simulink model "LQR_Model"  (R2023b)
settings: Solver=VariableStepAuto  StartTime=0.0  StopTime=10.0  RelTol=1e-3
values from neighbouring files (symbols this model uses):
  A_mat = [0 0 1 0;0 0 0 1;0 (b*d)/(E) (-(c*G)/E) 0 ; 0 ((a*d)/E) (-b*G)/E 0 ]    [LQR.m]    (also in matlab.mat = [0 0 0 0 0 0 16.4102446308 112.769220168 1 0 2.36879708342 2)
  B_mat = [0;0;(c)*(H);(b)*(H)]    [LQR.m]    (also in matlab.mat = [0 0 152.465167276 137.218650549])
  C_mat = [1 0 0 0 ; 0 1 0 0]    [LQR.m]    (also in matlab.mat = [1  0  0  0; 0  1  0  0])
  k = lqr(A_mat,B_mat,Q,R)    [LQR.m]    (also in matlab.mat = [-0.316227766017 614.603053164 -26.5092676997 65.1532424468])
settings Model: Creator=peter  LastModifiedBy=peter

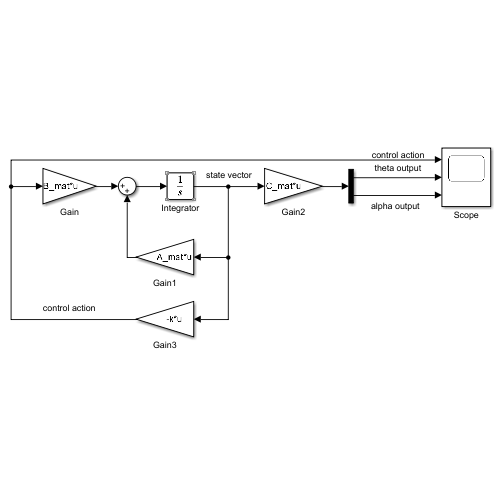
[thumbnail: Simulink's stored preview of the top-level diagram]
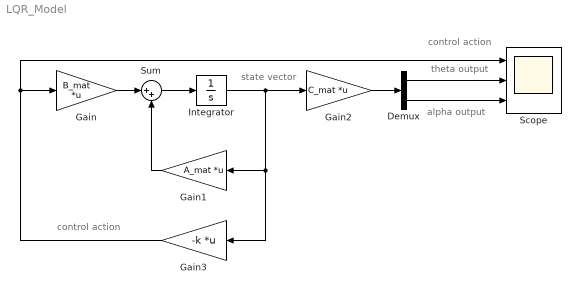
== system LQR_Model ==
  note: control action
  note: theta output
  note: alpha output
  note: state vector
  note: control action
  Demux : Demux  Outputs=2
  Gain : Gain  Gain=B_mat  Multiplication=Matrix(K*u)
  Gain1 : Gain  Gain=A_mat  Multiplication=Matrix(K*u)
  Gain2 : Gain  Gain=C_mat  Multiplication=Matrix(K*u)
  Gain3 : Gain  Gain=-k  Multiplication=Matrix(K*u)
  Integrator : Integrator  InitialCondition=[0.5 0.436 0 0]
  Scope : Scope  NumInputPorts=3
  Sum : Sum  Inputs=|++
  wires:
  Gain/1 -> Sum/1
  Sum/1 -> Integrator/1
  Integrator/1 -> Gain3/1, Gain1/1, Gain2/1
  Gain1/1 -> Sum/2
  Gain3/1 -> Gain/1, Scope/1
  Gain2/1 -> Demux/1
  Demux/1 -> Scope/2
  Demux/2 -> Scope/3
